simulink model "examples_of_mux_and_demux_block"  (R2021a)
settings: Solver=VariableStepAuto  StartTime=0.0  StopTime=1  RelTol=1e-3
settings Model: Creator=YasserNet  LastModifiedBy=YasserNet

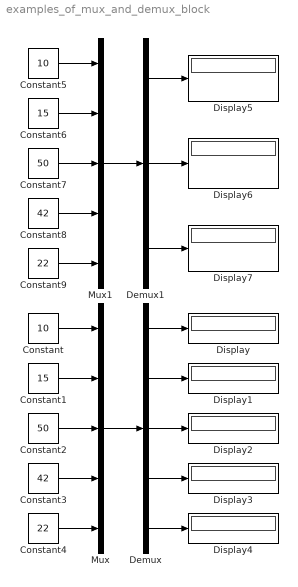
== system examples_of_mux_and_demux_block ==
  Constant : Constant  Value=10
  Constant1 : Constant  Value=15
  Constant2 : Constant  Value=50
  Constant3 : Constant  Value=42
  Constant4 : Constant  Value=22
  Constant5 : Constant  Value=10
  Constant6 : Constant  Value=15
  Constant7 : Constant  Value=50
  Constant8 : Constant  Value=42
  Constant9 : Constant  Value=22
  Demux : Demux  Outputs=5
  Demux1 : Demux  Outputs=3
  Display{,1..7} (8 alike) : Display
  Mux : Mux  Inputs=5
  Mux1 : Mux  Inputs=5
  wires:
  Demux/5 -> Display4/1
  Mux/1 -> Demux/1
  Demux/3 -> Display2/1
  Demux/4 -> Display3/1
  Demux/2 -> Display1/1
  Demux/1 -> Display/1
  Constant3/1 -> Mux/4
  Constant4/1 -> Mux/5
  Constant2/1 -> Mux/3
  Constant/1 -> Mux/1
  Mux1/1 -> Demux1/1
  Constant5/1 -> Mux1/1
  Constant9/1 -> Mux1/5
  Constant7/1 -> Mux1/3
  Demux1/1 -> Display5/1
  Constant1/1 -> Mux/2
  Demux1/2 -> Display6/1
  Constant8/1 -> Mux1/4
  Constant6/1 -> Mux1/2
  Demux1/3 -> Display7/1
